simulink model "piezobalken"  (R2016a)
settings: Solver=ode3  StartTime=0.0  StopTime=10  FixedStep=Ts  RelTol=1e-3
PostLoadFcn:
  | try
  | if isempty(which('ZHAWcbfcn'));
  | callback_fid07124=fopen('ZHAWcbfcn.m','w');
  | [~]=fprintf(callback_fid07124,'%s',get_param([bdroot,'/ Setup SLDRT'],'ClipboardFcn'));
  | [~]=fclose(callback_fid07124);
  | setpref('ZHAW_SLDRT_lib','cb_fcn',which('ZHAWcbfcn'))
  | clear callback_fid07124
  | end
  | catch
  | clear callback_fid07124
  | end
  | Ts=eval(get_param([bdroot,'/ Setup SLDRT'],'Ts'));
InitFcn:
  | Ts=eval(get_param([bdroot,'/ Setup SLDRT'],'Ts'));
undefined symbols (not defined in the file or in its folder): National_Instruments, PCIe
libraries: sldrtlib x3, simulink x1
(part 2 of 2)

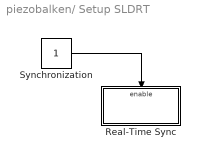
== system piezobalken/ Setup SLDRT ==
  Real-Time Sync : Subsystem
  Synchronization : Constant
  wires:
  Synchronization/1 -> Real-Time Sync/Enable

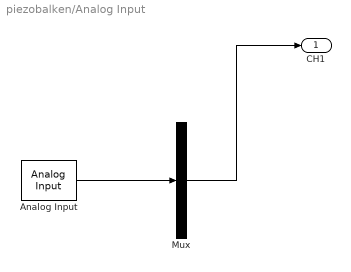
== system piezobalken/Analog Input ==
  Analog Input : sldrtlib/Analog Input  SampleTime=Ts  MaxMissedTicks=10  ShowMissedTicks=off  YieldWhenWaiting=off  DrvName=National_Instruments/PCIe-6321  DrvAddress=4294967295  DrvOptions="[1  0  0  2  2  2  2]"  Channels=ch_list  RangeMode=1  VoltRange=1  DataType=1
      settings: AttributesFormatString=National Instruments\nPCIe-6321 [auto]
  Mux : Demux  Outputs=1
  CH1 : Outport
  wires:
  Mux/1 -> CH1/1
  Analog Input/1 -> Mux/1

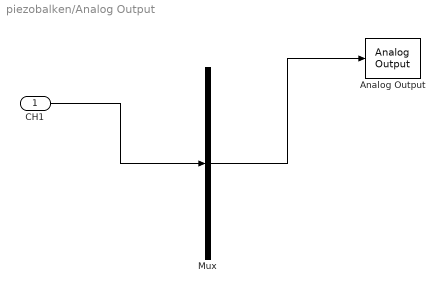
== system piezobalken/Analog Output ==
  CH1 : Inport
  Analog Output : sldrtlib/Analog Output  SampleTime=Ts  MaxMissedTicks=10  ShowMissedTicks=off  YieldWhenWaiting=off  DrvName=National_Instruments/PCIe-6321  DrvAddress=4294967295  DrvOptions="[1  0  0  2  2  2  2]"  Channels=ch_list  RangeMode=1  VoltRange=1  InitialValue=0  FinalValue=0
      settings: AttributesFormatString=National Instruments\nPCIe-6321 [auto]
  Mux : Mux  Inputs=1
  wires:
  Mux/1 -> Analog Output/1
  CH1/1 -> Mux/1

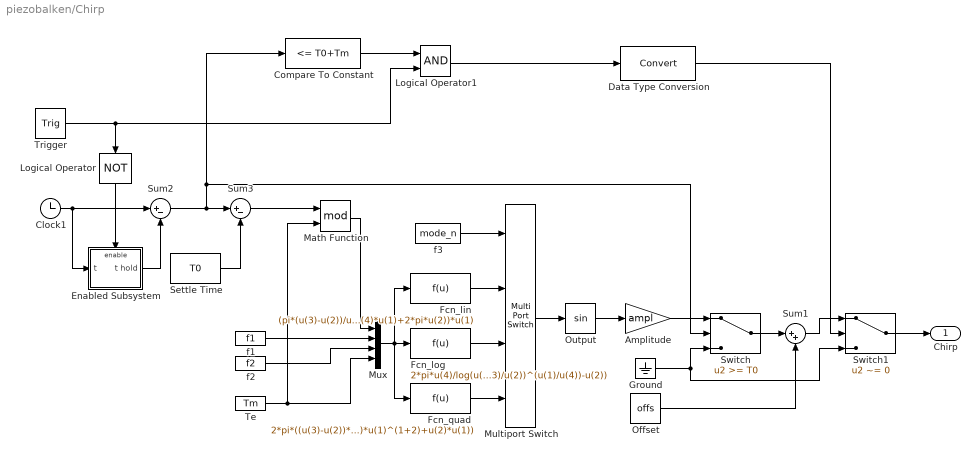
== system piezobalken/Chirp ==
  Amplitude : Gain  Gain=ampl
  Clock1 : Clock
      settings: DisableCoverage=on
  Compare To Constant : simulink/Logic and Bit Operations/Compare To Constant  relop=<=  const=T0+Tm  OutDataTypeStr=boolean
  Data Type Conversion : DataTypeConversion
  Enabled Subsystem : Subsystem  TreatAsAtomicUnit=on
  Fcn_lin : Fcn  Expr=(pi*(u(3)-u(2))/u(4)*u(1)+2*pi*u(2))*u(1)
  Fcn_log : Fcn  Expr=2*pi*u(4)/log(u(3)/u(2))*(u(2)*(u(3)/u(2))^(u(1)/u(4))-u(2))
  Fcn_quad : Fcn  Expr=2*pi*((u(3)-u(2))*u(4)^(-2)/(1+2)*u(1)^(1+2)+u(2)*u(1))
  Ground : Ground
  Logical Operator : Logic  Operator=NOT  AllPortsSameDT=off  OutDataTypeStr=boolean
  Logical Operator1 : Logic  AllPortsSameDT=off  OutDataTypeStr=boolean
  Math Function : Math  Operator=mod  SaturateOnIntegerOverflow=on
  Multiport Switch : MultiPortSwitch
  Mux : Mux
  Offset : Constant  Value=offs
  Output : Trigonometry
  Settle Time : Constant  Value=T0
  Sum1 : Sum  Inputs=|++
  Sum2 : Sum  Inputs=|+-
  Sum3 : Sum  Inputs=|+-
  Switch : Switch  Threshold=T0
  Switch1 : Switch  Criteria=u2 ~= 0
  Te : Constant  Value=Tm
  Trigger : Constant  Value=Trig
  f1 : Constant  Value=f1
  f2 : Constant  Value=f2
  f3 : Constant  Value=mode_n
  Chirp : Outport
  wires:
  Data Type Conversion/1 -> Switch1/2
  Logical Operator1/1 -> Data Type Conversion/1
  Compare To Constant/1 -> Logical Operator1/1
  Sum1/1 -> Switch1/1
  Switch1/1 -> Chirp/1
  Sum2/1 -> Sum3/1, Compare To Constant/1, Switch/2
  Settle Time/1 -> Sum3/2
  Ground/1 -> Switch1/3, Switch/3
  Amplitude/1 -> Switch/1
  Switch/1 -> Sum1/1
  Te/1 -> Math Function/2, Mux/4
  Sum3/1 -> Math Function/1
  Offset/1 -> Sum1/2
  Output/1 -> Amplitude/1
  Clock1/1 -> Enabled Subsystem/1(t), Sum2/1
  Mux/1 -> Fcn_quad/1, Fcn_lin/1, Fcn_log/1
  f1/1 -> Mux/2
  f2/1 -> Mux/3
  Math Function/1 -> Mux/1
  Multiport Switch/1 -> Output/1
  Fcn_quad/1 -> Multiport Switch/4
  Fcn_log/1 -> Multiport Switch/3
  Fcn_lin/1 -> Multiport Switch/2
  f3/1 -> Multiport Switch/1
  Trigger/1 -> Logical Operator/1, Logical Operator1/2
  Enabled Subsystem/1(t hold) -> Sum2/2
  Logical Operator/1 -> Enabled Subsystem/Enable

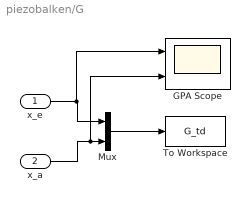
== system piezobalken/G ==
  x_e : Inport
  x_a : Inport  Port=2
  GPA Scope : Scope  NumInputPorts=2
      settings: CopyFcn=try ZHAWcbfcn('copyScope'); end  NameChangeFcn=try ZHAWcbfcn('namechangeScope'); end
  Mux : Mux  Inputs=2
  To Workspace : ToWorkspace  VariableName=G_td  SaveFormat=Structure With Time  SampleTime=Ts
  wires:
  Mux/1 -> To Workspace/1
  x_a/1 -> Mux/2, GPA Scope/2
  x_e/1 -> Mux/1, GPA Scope/1

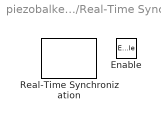
== system piezobalken/ Setup SLDRT/Real-Time Sync ==
  Enable : EnablePort
  Real-Time Synchronization : sldrtlib/Real-Time Synchronization  SampleTime=Ts  MaxMissedTicks=inf  ShowMissedTicks=off  YieldWhenWaiting=off

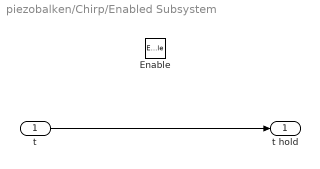
== system piezobalken/Chirp/Enabled Subsystem ==
  t : Inport
  Enable : EnablePort
  t hold : Outport
  wires:
  t/1 -> t hold/1
